simulink model "Exp_4_4"  (R2024b)
settings: Solver=VariableStepAuto  StartTime=0.0  StopTime=15  RelTol=1e-3
settings Model: Creator=Rj Avro Biswas  LastModifiedBy=Rj Avro Biswas

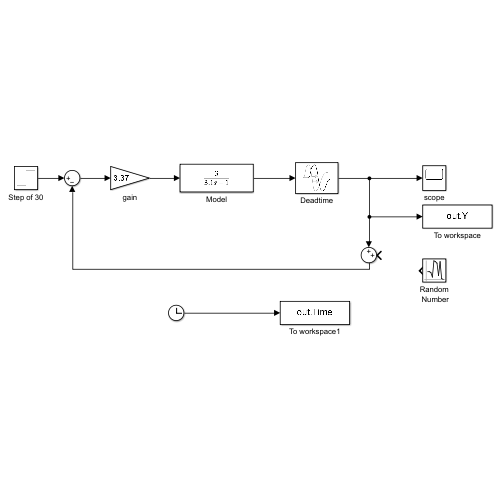
[thumbnail: Simulink's stored preview of the top-level diagram]
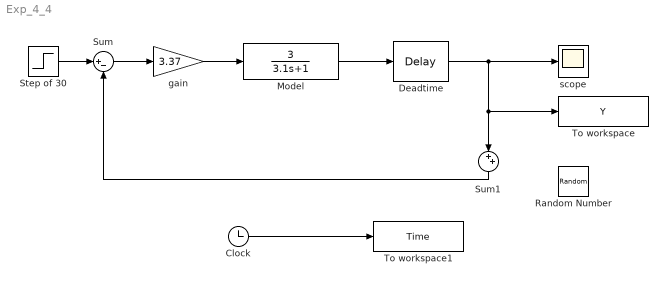
== system Exp_4_4 ==
  Clock : Clock
  Deadtime : TransportDelay  DelayTime=.15*5/60
  Model : TransferFcn  Numerator=3  Denominator=[3.1 1]
  Random Number : RandomNumber  Variance=0.5  Seed=61233  SampleTime=0
  Step of 30 : Step  Time=0  After=30  SampleTime=0
  Sum : Sum  Inputs=|+-
  Sum1 : Sum  Inputs=|++
  To workspace : ToWorkspace  VariableName=Y  SaveFormat=Structure  SampleTime=-1
  To workspace1 : ToWorkspace  VariableName=Time  SaveFormat=Structure  SampleTime=-1
  gain : Gain  Gain=3.37
  scope : Scope
  wires:
  Step of 30/1 -> Sum/1
  Sum/1 -> gain/1
  gain/1 -> Model/1
  Model/1 -> Deadtime/1
  Sum1/1 -> Sum/2
  Deadtime/1 -> To workspace/1, Sum1/1, scope/1
  Clock/1 -> To workspace1/1
